simulink model "vd_controller_E9"  (R2017b)
settings: configuration reference "E9_ECU_Configuration" (kept outside this file)
undefined symbols (not defined in the file or in its folder): activate_TC_forMinimal_pTC, ConstantSlipPercent_XCP_pTC, DifferentTorqueFrontAxis_tc, disable_9D_front, disable_9D_rear, disable_slipanglesensor, DiscIntNeverNeededParam, Fz0, lambda_mux_switch_over_XCP_pTC, lambda_mux_XCP_pTC, Lyap_kp_switch_over_XCP_pTC, Lyap_kp_XCP_pTC, Lyap_p, Lyap_TCint, LyapDiscFilter, lyapFilterCoeff_switch_over_XCP_pTC, lyapFilterCoeff_XCP_pTC, mask_SelectInput_pGL, p_Dx1, p_Dx2, Slip_switch_over_XCP_pTC, Sq_PosBadGradient, Sq_PosIsFrozen, Sq_PosOutOfBounds, tire_r_dyn, velLimitInput_switch_over_XCP_pTC, velLimitInput_XCP_pTC, WheelInertia
libraries: SignalProcessingLib x37, simulink x30, hdlsllib x3
(part 2 of 2)

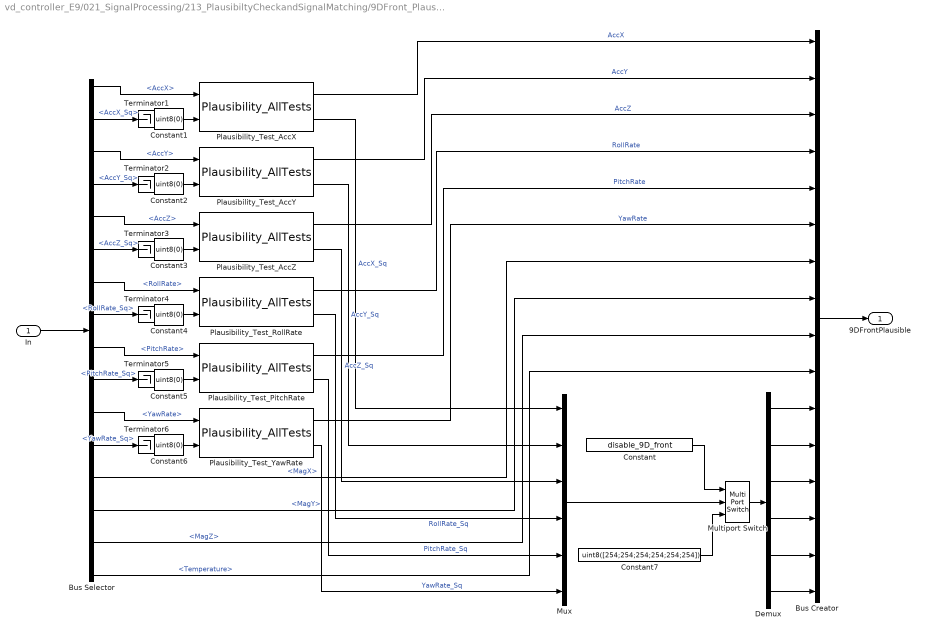
== system vd_controller_E9/021_SignalProcessing/213_PlausibiltyCheckandSignalMatching/9DFront_Plausibility ==
  In : Inport  OutDataTypeStr=Bus: control_9D
  Bus Creator : BusCreator  Inputs=16  OutDataTypeStr=Bus: control_9D
  Bus Selector : BusSelector  OutputSignals=AccX,AccX_Sq,AccY,AccY_Sq,AccZ,AccZ_Sq,RollRate,RollRate_Sq,PitchRate,PitchRate_Sq,YawRate,YawRate_Sq,MagX,MagY,MagZ,Temperature
  Constant : Constant  Value=disable_9D_front
  Constant{1..6} (6 alike) : Constant  Value=uint8(0)
  Constant7 : Constant  Value=uint8([254;254;254;254;254;254])
  Demux : Demux  Outputs=6
  Multiport Switch : MultiPortSwitch  DataPortOrder=Zero-based contiguous  Inputs=2
  Mux : Mux  Inputs=6
  Plausibility_Test_AccX : SignalProcessingLib/Plausibility_AllTests  alpha=0.3  checkGradient=off  deviation=0  threshold=0  alpha2=0  increasingPercentage=0  signalBounds=1e-8  stepDelay=25  upperBound=50  lowerBound=-50  useAlternativeValue=off  useManualAlternativeValue=off  manualAlternativeValue=0
  Plausibility_Test_AccY : SignalProcessingLib/Plausibility_AllTests  alpha=0.3  checkGradient=off  deviation=0  threshold=0  alpha2=0  increasingPercentage=0  signalBounds=1e-8  stepDelay=25  upperBound=50  lowerBound=-50  useAlternativeValue=off  useManualAlternativeValue=off  manualAlternativeValue=0
  Plausibility_Test_AccZ : SignalProcessingLib/Plausibility_AllTests  alpha=0.3  checkGradient=off  deviation=0  threshold=0  alpha2=0  increasingPercentage=0  signalBounds=1e-8  stepDelay=25  upperBound=50  lowerBound=-50  useAlternativeValue=off  useManualAlternativeValue=off  manualAlternativeValue=0
  Plausibility_Test_PitchRate : SignalProcessingLib/Plausibility_AllTests  alpha=0.3  checkGradient=off  deviation=0  threshold=0  alpha2=0  increasingPercentage=0  signalBounds=1e-8  stepDelay=25  upperBound=1.6  lowerBound=-1.6  useAlternativeValue=off  useManualAlternativeValue=off  manualAlternativeValue=0
  Plausibility_Test_RollRate : SignalProcessingLib/Plausibility_AllTests  alpha=0.3  checkGradient=off  deviation=0  threshold=0  alpha2=0  increasingPercentage=0  signalBounds=1e-8  stepDelay=25  upperBound=1.6  lowerBound=-1.6  useAlternativeValue=off  useManualAlternativeValue=off  manualAlternativeValue=0
  Plausibility_Test_YawRate : SignalProcessingLib/Plausibility_AllTests  alpha=0.3  checkGradient=off  deviation=0  threshold=0  alpha2=0  increasingPercentage=0  signalBounds=1e-8  stepDelay=25  upperBound=3  lowerBound=-3  useAlternativeValue=off  useManualAlternativeValue=off  manualAlternativeValue=0
  Terminator{1..6} (6 alike) : Terminator
  9DFrontPlausible : Outport
  wires:
  Plausibility_Test_AccY/1 -> Bus Creator/2  "AccY"
  Bus Selector/3 -> Plausibility_Test_AccY/1  "<AccY>"
  In/1 -> Bus Selector/1
  Plausibility_Test_AccX/1 -> Bus Creator/1  "AccX"
  Bus Selector/1 -> Plausibility_Test_AccX/1  "<AccX>"
  Plausibility_Test_AccZ/1 -> Bus Creator/3  "AccZ"
  Bus Selector/5 -> Plausibility_Test_AccZ/1  "<AccZ>"
  Bus Selector/7 -> Plausibility_Test_RollRate/1  "<RollRate>"
  Plausibility_Test_RollRate/1 -> Bus Creator/4  "RollRate"
  Bus Creator/1 -> 9DFrontPlausible/1
  Plausibility_Test_PitchRate/1 -> Bus Creator/5  "PitchRate"
  Plausibility_Test_YawRate/1 -> Bus Creator/6  "YawRate"
  Bus Selector/9 -> Plausibility_Test_PitchRate/1  "<PitchRate>"
  Bus Selector/11 -> Plausibility_Test_YawRate/1  "<YawRate>"
  Plausibility_Test_YawRate/2 -> Mux/6  "YawRate_Sq"
  Plausibility_Test_PitchRate/2 -> Mux/5  "PitchRate_Sq"
  Plausibility_Test_RollRate/2 -> Mux/4  "RollRate_Sq"
  Plausibility_Test_AccZ/2 -> Mux/3  "AccZ_Sq"
  Bus Selector/13 -> Bus Creator/7  "<MagX>"
  Bus Selector/14 -> Bus Creator/8  "<MagY>"
  Bus Selector/15 -> Bus Creator/9  "<MagZ>"
  Bus Selector/16 -> Bus Creator/10  "<Temperature>"
  Plausibility_Test_AccX/2 -> Mux/1  "AccX_Sq"
  Plausibility_Test_AccY/2 -> Mux/2  "AccY_Sq"
  Constant1/1 -> Plausibility_Test_AccX/2
  Bus Selector/2 -> Terminator1/1  "<AccX_Sq>"
  Constant2/1 -> Plausibility_Test_AccY/2
  Bus Selector/4 -> Terminator2/1  "<AccY_Sq>"
  Constant3/1 -> Plausibility_Test_AccZ/2
  Bus Selector/6 -> Terminator3/1  "<AccZ_Sq>"
  Constant4/1 -> Plausibility_Test_RollRate/2
  Bus Selector/8 -> Terminator4/1  "<RollRate_Sq>"
  Constant5/1 -> Plausibility_Test_PitchRate/2
  Bus Selector/10 -> Terminator5/1  "<PitchRate_Sq>"
  Constant6/1 -> Plausibility_Test_YawRate/2
  Bus Selector/12 -> Terminator6/1  "<YawRate_Sq>"
  Mux/1 -> Multiport Switch/2
  Constant7/1 -> Multiport Switch/3
  Multiport Switch/1 -> Demux/1
  Constant/1 -> Multiport Switch/1
  Demux/1 -> Bus Creator/11
  Demux/2 -> Bus Creator/12
  Demux/3 -> Bus Creator/13
  Demux/4 -> Bus Creator/14
  Demux/5 -> Bus Creator/15
  Demux/6 -> Bus Creator/16

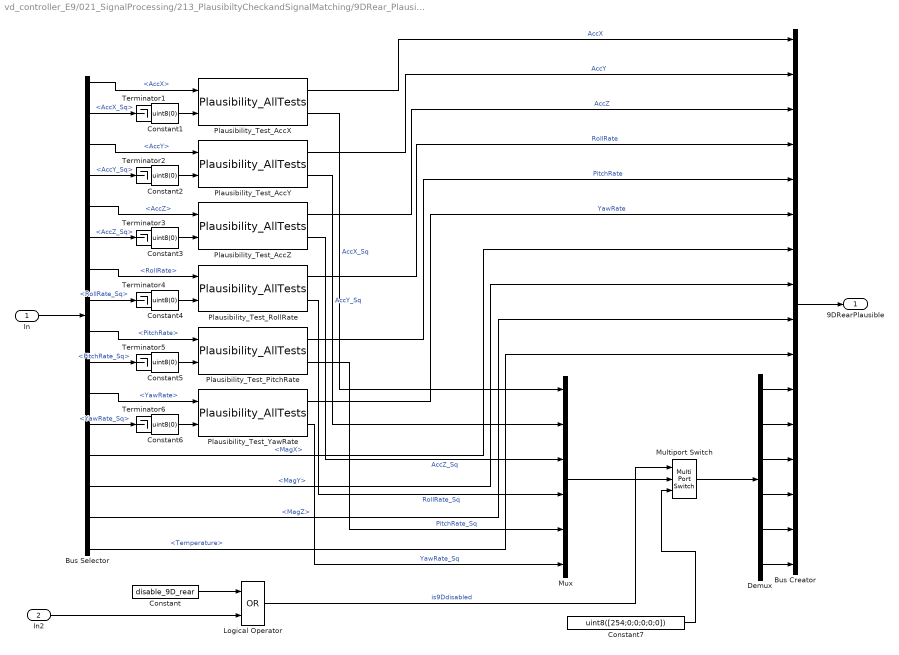
== system vd_controller_E9/021_SignalProcessing/213_PlausibiltyCheckandSignalMatching/9DRear_Plausibility ==
  In : Inport  OutDataTypeStr=Bus: control_9D
  In2 : Inport  Port=2
  Bus Creator : BusCreator  Inputs=16  OutDataTypeStr=Bus: control_9D
  Bus Selector : BusSelector  OutputSignals=AccX,AccX_Sq,AccY,AccY_Sq,AccZ,AccZ_Sq,RollRate,RollRate_Sq,PitchRate,PitchRate_Sq,YawRate,YawRate_Sq,MagX,MagY,MagZ,Temperature
  Constant : Constant  Value=disable_9D_rear
  Constant{1..6} (6 alike) : Constant  Value=uint8(0)
  Constant7 : Constant  Value=uint8([254;0;0;0;0;0])
  Demux : Demux  Outputs=6
  Logical Operator : Logic  Operator=OR  AllPortsSameDT=off  OutDataTypeStr=boolean
  Multiport Switch : MultiPortSwitch  DataPortOrder=Zero-based contiguous  Inputs=2
  Mux : Mux  Inputs=6
  Plausibility_Test_AccX : SignalProcessingLib/Plausibility_AllTests  alpha=0.3  checkGradient=off  deviation=0  threshold=0  alpha2=0  increasingPercentage=0  signalBounds=1e-8  stepDelay=25  upperBound=50  lowerBound=-50  useAlternativeValue=off  useManualAlternativeValue=off  manualAlternativeValue=0
  Plausibility_Test_AccY : SignalProcessingLib/Plausibility_AllTests  alpha=0.3  checkGradient=off  deviation=0  threshold=0  alpha2=0  increasingPercentage=0  signalBounds=1e-8  stepDelay=25  upperBound=50  lowerBound=-50  useAlternativeValue=off  useManualAlternativeValue=off  manualAlternativeValue=0
  Plausibility_Test_AccZ : SignalProcessingLib/Plausibility_AllTests  alpha=0.3  checkGradient=off  deviation=0  threshold=0  alpha2=0  increasingPercentage=0  signalBounds=1e-8  stepDelay=25  upperBound=50  lowerBound=-50  useAlternativeValue=off  useManualAlternativeValue=off  manualAlternativeValue=0
  Plausibility_Test_PitchRate : SignalProcessingLib/Plausibility_AllTests  alpha=0.3  checkGradient=off  deviation=0  threshold=0  alpha2=0  increasingPercentage=0  signalBounds=1e-8  stepDelay=25  upperBound=1.6  lowerBound=-1.6  useAlternativeValue=off  useManualAlternativeValue=off  manualAlternativeValue=0
  Plausibility_Test_RollRate : SignalProcessingLib/Plausibility_AllTests  alpha=0.3  checkGradient=off  deviation=0  threshold=0  alpha2=0  increasingPercentage=0  signalBounds=1e-8  stepDelay=25  upperBound=1.6  lowerBound=-1.6  useAlternativeValue=off  useManualAlternativeValue=off  manualAlternativeValue=0
  Plausibility_Test_YawRate : SignalProcessingLib/Plausibility_AllTests  alpha=0.3  checkGradient=off  deviation=0  threshold=0  alpha2=0  increasingPercentage=0  signalBounds=1e-8  stepDelay=25  upperBound=3  lowerBound=-3  useAlternativeValue=off  useManualAlternativeValue=off  manualAlternativeValue=0
  Terminator{1..6} (6 alike) : Terminator
  9DRearPlausible : Outport
  wires:
  Plausibility_Test_AccY/1 -> Bus Creator/2  "AccY"
  Bus Selector/16 -> Bus Creator/10  "<Temperature>"
  Bus Selector/13 -> Bus Creator/7  "<MagX>"
  Plausibility_Test_YawRate/1 -> Bus Creator/6  "YawRate"
  Bus Selector/15 -> Bus Creator/9  "<MagZ>"
  Plausibility_Test_RollRate/1 -> Bus Creator/4  "RollRate"
  Bus Creator/1 -> 9DRearPlausible/1
  Bus Selector/7 -> Plausibility_Test_RollRate/1  "<RollRate>"
  Bus Selector/5 -> Plausibility_Test_AccZ/1  "<AccZ>"
  Bus Selector/11 -> Plausibility_Test_YawRate/1  "<YawRate>"
  In/1 -> Bus Selector/1
  Plausibility_Test_AccZ/1 -> Bus Creator/3  "AccZ"
  Plausibility_Test_PitchRate/1 -> Bus Creator/5  "PitchRate"
  Plausibility_Test_AccX/1 -> Bus Creator/1  "AccX"
  Bus Selector/1 -> Plausibility_Test_AccX/1  "<AccX>"
  Bus Selector/3 -> Plausibility_Test_AccY/1  "<AccY>"
  Bus Selector/2 -> Terminator1/1  "<AccX_Sq>"
  Plausibility_Test_AccZ/2 -> Mux/3  "AccZ_Sq"
  Plausibility_Test_AccY/2 -> Mux/2  "AccY_Sq"
  Plausibility_Test_PitchRate/2 -> Mux/5  "PitchRate_Sq"
  Bus Selector/14 -> Bus Creator/8  "<MagY>"
  Plausibility_Test_AccX/2 -> Mux/1  "AccX_Sq"
  Plausibility_Test_YawRate/2 -> Mux/6  "YawRate_Sq"
  Plausibility_Test_RollRate/2 -> Mux/4  "RollRate_Sq"
  Bus Selector/9 -> Plausibility_Test_PitchRate/1  "<PitchRate>"
  Constant1/1 -> Plausibility_Test_AccX/2
  Constant2/1 -> Plausibility_Test_AccY/2
  Bus Selector/4 -> Terminator2/1  "<AccY_Sq>"
  Constant3/1 -> Plausibility_Test_AccZ/2
  Bus Selector/6 -> Terminator3/1  "<AccZ_Sq>"
  Constant4/1 -> Plausibility_Test_RollRate/2
  Bus Selector/8 -> Terminator4/1  "<RollRate_Sq>"
  Constant5/1 -> Plausibility_Test_PitchRate/2
  Bus Selector/10 -> Terminator5/1  "<PitchRate_Sq>"
  Constant6/1 -> Plausibility_Test_YawRate/2
  Bus Selector/12 -> Terminator6/1  "<YawRate_Sq>"
  Constant7/1 -> Multiport Switch/3
  Constant/1 -> Logical Operator/1
  Mux/1 -> Multiport Switch/2
  Multiport Switch/1 -> Demux/1
  Demux/6 -> Bus Creator/16
  Demux/5 -> Bus Creator/15
  Demux/4 -> Bus Creator/14
  Demux/3 -> Bus Creator/13
  Demux/2 -> Bus Creator/12
  Demux/1 -> Bus Creator/11
  Logical Operator/1 -> Multiport Switch/1  "is9Ddisabled"
  In2/1 -> Logical Operator/2

== system vd_controller_E9/021_SignalProcessing/213_PlausibiltyCheckandSignalMatching/DriverInput ==
  note: Der DrivingMode aus Inport 2 ist der, der beim Start ausgewählr wurde. Dieser wurde beim E9 in dem Block InverterInControl bestimmt und lässt sich während der Fahrt nicht ändern. Früher in die Funktionsstruktur integreireren, da so weniger umständlich.
  DriverInput_in : Inport
  DrivingMode : Inport  Port=2
  Bus Creator : BusCreator  Inputs=9
  Bus Selector : BusSelector  OutputSignals=db_PTM,db_button_low,vd_button_1,vd_button_2,vd_turnbutton_1,vd_turnbutton_2,driver,DriverInput_Sq
  DriverInput : Outport
  wires:
  DriverInput_in/1 -> Bus Selector/1
  Bus Creator/1 -> DriverInput/1  "DriverInput"
  Bus Selector/1 -> Bus Creator/1  "<db_PTM>"
  Bus Selector/2 -> Bus Creator/2  "<db_button_low>"
  Bus Selector/3 -> Bus Creator/3  "<vd_button_1>"
  Bus Selector/4 -> Bus Creator/4  "<vd_button_2>"
  Bus Selector/5 -> Bus Creator/5  "<vd_turnbutton_1>"
  Bus Selector/6 -> Bus Creator/6  "<vd_turnbutton_2>"
  Bus Selector/7 -> Bus Creator/7  "<driver>"
  DrivingMode/1 -> Bus Creator/9
  Bus Selector/8 -> Bus Creator/8  "<DriverInput_Sq>"

== system vd_controller_E9/021_SignalProcessing/213_PlausibiltyCheckandSignalMatching/DriverRequest_Plausibility ==
  In : Inport  OutDataTypeStr=Bus: control_DriverRequest
  Bus Creator : BusCreator  Inputs=11  OutDataTypeStr=Bus: control_DriverRequest
      settings: InheritFromInputs=off
  Bus Selector : BusSelector  OutputSignals=Pedal_BrakeMech_Value,Pedal_BrakeRecu_Value,SteeringwheelAngle,Pedal_Accel_Value,Pedal_TorqueValid_flag,Pedal_BrakeHard_flag,Pedal_BrakeMech_flag,SteeringValid_flag,Pedal_BrakeValid_flag,SteeringwheelAngle_Sq,Pedal_Accel_Value_Sq
  Data Type Conversion{1..3,6} (4 alike) : DataTypeConversion  OutDataTypeStr=uint8
  Data Type Conversion{4..5,7,9} (4 alike) : DataTypeConversion  OutDataTypeStr=single
  Plausibility_Test_AcceleratorPedal : SignalProcessingLib/Plausibility_AllTests  alpha=0.3  checkGradient=off  deviation=0  threshold=0  alpha2=0  increasingPercentage=0  signalBounds=1e-10  stepDelay=40  upperBound=1  lowerBound=0  useAlternativeValue=off  useManualAlternativeValue=off  manualAlternativeValue=0
  Plausibility_Test_SteeringwheelAngle : SignalProcessingLib/Plausibility_AllTests  alpha=0.3  checkGradient=off  deviation=0  threshold=0  alpha2=0  increasingPercentage=0  signalBounds=1e-10  stepDelay=40  upperBound=120  lowerBound=-120  useAlternativeValue=off  useManualAlternativeValue=off  manualAlternativeValue=0
  DriverRequest : Outport
  wires:
  In/1 -> Bus Selector/1
  Bus Creator/1 -> DriverRequest/1
  Bus Selector/1 -> Data Type Conversion7/1  "<Pedal_BrakeMech_Value>"
  Bus Selector/2 -> Data Type Conversion5/1  "<Pedal_BrakeRecu_Value>"
  Bus Selector/3 -> Plausibility_Test_SteeringwheelAngle/1  "<SteeringwheelAngle>"
  Plausibility_Test_SteeringwheelAngle/1 -> Data Type Conversion4/1  "SteeringwheelAngle"
  Bus Selector/4 -> Plausibility_Test_AcceleratorPedal/1  "<Pedal_Accel_Value>"
  Bus Selector/5 -> Bus Creator/5  "<Pedal_TorqueValid_flag>"
  Bus Selector/6 -> Bus Creator/6  "<Pedal_BrakeHard_flag>"
  Bus Selector/7 -> Bus Creator/7  "<Pedal_BrakeMech_flag>"
  Bus Selector/8 -> Bus Creator/8  "<SteeringValid_flag>"
  Bus Selector/9 -> Bus Creator/9  "<Pedal_BrakeValid_flag>"
  Plausibility_Test_SteeringwheelAngle/2 -> Data Type Conversion3/1  "SteeringwheelAngle_Sq"
  Plausibility_Test_AcceleratorPedal/1 -> Data Type Conversion9/1  "Pedal_Accel_Value"
  Bus Selector/10 -> Data Type Conversion6/1  "<SteeringwheelAngle_Sq>"
  Data Type Conversion7/1 -> Bus Creator/1
  Data Type Conversion5/1 -> Bus Creator/2
  Data Type Conversion4/1 -> Bus Creator/3
  Data Type Conversion9/1 -> Bus Creator/4
  Bus Selector/11 -> Data Type Conversion1/1  "<Pedal_Accel_Value_Sq>"
  Plausibility_Test_AcceleratorPedal/2 -> Data Type Conversion2/1  "Pedal_Accel_Value_Sq"
  Data Type Conversion2/1 -> Bus Creator/11
  Data Type Conversion6/1 -> Plausibility_Test_SteeringwheelAngle/2
  Data Type Conversion1/1 -> Plausibility_Test_AcceleratorPedal/2
  Data Type Conversion3/1 -> Bus Creator/10

== system vd_controller_E9/021_SignalProcessing/213_PlausibiltyCheckandSignalMatching/Electric_Plausibility ==
  In : Inport  OutDataTypeStr=Bus: control_Electric
  Bus Creator : BusCreator  Inputs=12  OutDataTypeStr=Bus: control_Electric
  Bus Selector : BusSelector  OutputSignals=BatSOC,BatVoltage,BatPower,BatCurrent,AvgCellVoltage,MaxCellVoltage,MinCellVoltage,IVTEnergy,MinCellTemp,IVT_VoltageCurrent_Sq,IVT_Energy_Sq,HVM_BMS_Sq
  Data Type Conversion22 : DataTypeConversion  OutDataTypeStr=single
  Plausibility_Test_IVTEnergy : SignalProcessingLib/Plausibility_AllTests  alpha=0.5  checkGradient=off  deviation=0  threshold=0  alpha2=0  increasingPercentage=0  signalBounds=1e-10  stepDelay=40  upperBound=120000  lowerBound=-120000  useAlternativeValue=off  useManualAlternativeValue=off  manualAlternativeValue=0
  ElectricPlausible : Outport
  wires:
  Bus Selector/8 -> Plausibility_Test_IVTEnergy/1  "<IVTEnergy>"
  Bus Selector/7 -> Bus Creator/7  "<MinCellVoltage>"
  In/1 -> Bus Selector/1
  Bus Creator/1 -> ElectricPlausible/1  "Electric"
  Bus Selector/1 -> Bus Creator/1  "<BatSOC>"
  Bus Selector/2 -> Bus Creator/2  "<BatVoltage>"
  Bus Selector/3 -> Bus Creator/3  "<BatPower>"
  Bus Selector/4 -> Bus Creator/4  "<BatCurrent>"
  Bus Selector/5 -> Bus Creator/5  "<AvgCellVoltage>"
  Bus Selector/6 -> Bus Creator/6  "<MaxCellVoltage>"
  Bus Selector/9 -> Bus Creator/9  "<MinCellTemp>"
  Bus Selector/10 -> Bus Creator/10  "<IVT_VoltageCurrent_Sq>"
  Bus Selector/11 -> Plausibility_Test_IVTEnergy/2  "<IVT_Energy_Sq>"
  Bus Selector/12 -> Bus Creator/12  "<HVM_BMS_Sq>"
  Plausibility_Test_IVTEnergy/2 -> Bus Creator/11  "IVTEnergy_Sq"
  Plausibility_Test_IVTEnergy/1 -> Data Type Conversion22/1  "IVTEnergy"
  Data Type Conversion22/1 -> Bus Creator/8

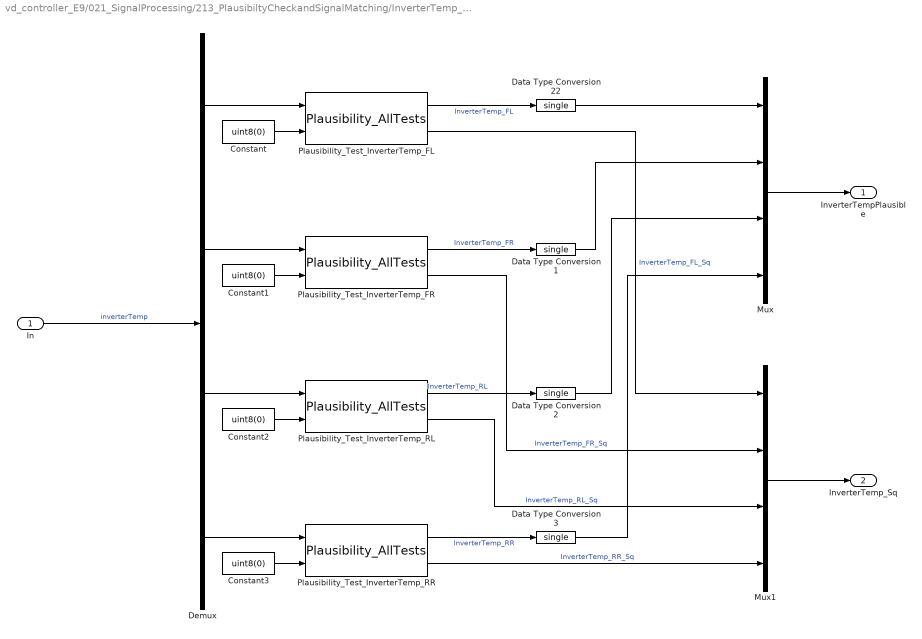
== system vd_controller_E9/021_SignalProcessing/213_PlausibiltyCheckandSignalMatching/InverterTemp_Plausibility ==
  In : Inport  OutDataTypeStr=single  PortDimensions=4
  Constant{,1..3} (4 alike) : Constant  Value=uint8(0)
  Data Type Conversion{1..3,22} (4 alike) : DataTypeConversion  OutDataTypeStr=single
  Demux : Demux
  Mux : Mux
  Mux1 : Mux
  Plausibility_Test_InverterTemp_FL : SignalProcessingLib/Plausibility_AllTests  alpha=0  checkGradient=off  deviation=0  threshold=0  alpha2=0  increasingPercentage=0  signalBounds=1e-12  stepDelay=40  upperBound=75  lowerBound=-10  useAlternativeValue=off  useManualAlternativeValue=off  manualAlternativeValue=0
  Plausibility_Test_InverterTemp_FR : SignalProcessingLib/Plausibility_AllTests  alpha=0.5  checkGradient=off  deviation=0  threshold=0  alpha2=0  increasingPercentage=0  signalBounds=1e-12  stepDelay=40  upperBound=75  lowerBound=-10  useAlternativeValue=off  useManualAlternativeValue=off  manualAlternativeValue=0
  Plausibility_Test_InverterTemp_RL : SignalProcessingLib/Plausibility_AllTests  alpha=0.5  checkGradient=off  deviation=0  threshold=0  alpha2=0  increasingPercentage=0  signalBounds=1e-12  stepDelay=40  upperBound=75  lowerBound=-10  useAlternativeValue=off  useManualAlternativeValue=off  manualAlternativeValue=0
  Plausibility_Test_InverterTemp_RR : SignalProcessingLib/Plausibility_AllTests  alpha=0.5  checkGradient=off  deviation=0  threshold=0  alpha2=0  increasingPercentage=0  signalBounds=1e-12  stepDelay=40  upperBound=75  lowerBound=-10  useAlternativeValue=off  useManualAlternativeValue=off  manualAlternativeValue=0
  InverterTempPlausible : Outport
  InverterTemp_Sq : Outport  Port=2
  wires:
  Plausibility_Test_InverterTemp_FR/1 -> Data Type Conversion1/1  "InverterTemp_FR"
  In/1 -> Demux/1  "inverterTemp"
  Plausibility_Test_InverterTemp_FL/1 -> Data Type Conversion22/1  "InverterTemp_FL"
  Plausibility_Test_InverterTemp_RL/1 -> Data Type Conversion2/1  "InverterTemp_RL"
  Demux/1 -> Plausibility_Test_InverterTemp_FL/1
  Demux/2 -> Plausibility_Test_InverterTemp_FR/1
  Demux/3 -> Plausibility_Test_InverterTemp_RL/1
  Plausibility_Test_InverterTemp_RL/2 -> Mux1/3  "InverterTemp_RL_Sq"
  Plausibility_Test_InverterTemp_FR/2 -> Mux1/2  "InverterTemp_FR_Sq"
  Demux/4 -> Plausibility_Test_InverterTemp_RR/1
  Constant/1 -> Plausibility_Test_InverterTemp_FL/2
  Constant1/1 -> Plausibility_Test_InverterTemp_FR/2
  Constant2/1 -> Plausibility_Test_InverterTemp_RL/2
  Constant3/1 -> Plausibility_Test_InverterTemp_RR/2
  Plausibility_Test_InverterTemp_RR/1 -> Data Type Conversion3/1  "InverterTemp_RR"
  Mux/1 -> InverterTempPlausible/1
  Mux1/1 -> InverterTemp_Sq/1
  Plausibility_Test_InverterTemp_RR/2 -> Mux1/4  "InverterTemp_RR_Sq"
  Plausibility_Test_InverterTemp_FL/2 -> Mux1/1  "InverterTemp_FL_Sq"
  Data Type Conversion22/1 -> Mux/1
  Data Type Conversion1/1 -> Mux/2
  Data Type Conversion2/1 -> Mux/3
  Data Type Conversion3/1 -> Mux/4

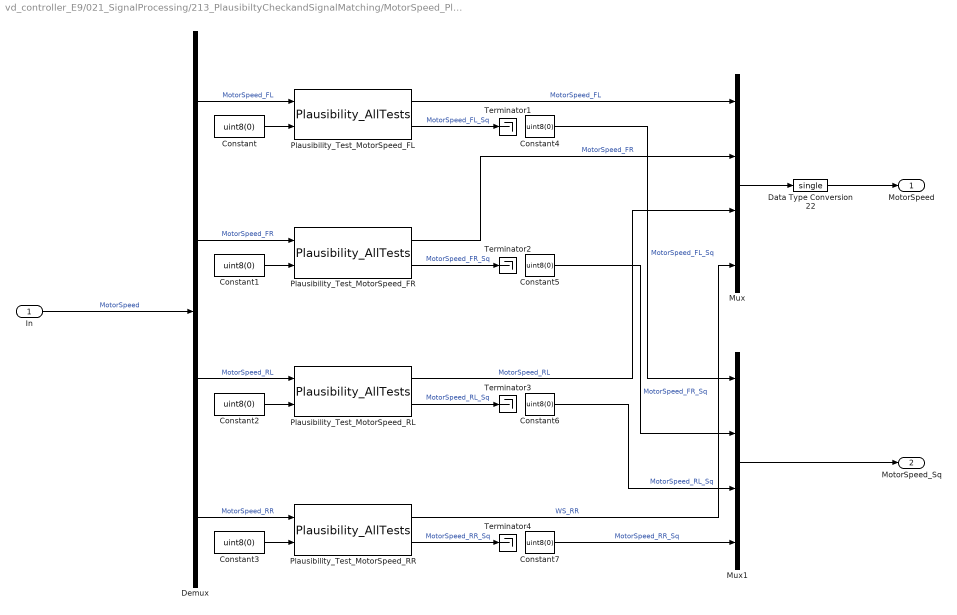
== system vd_controller_E9/021_SignalProcessing/213_PlausibiltyCheckandSignalMatching/MotorSpeed_Plausibility ==
  In : Inport
  Constant{,1..7} (8 alike) : Constant  Value=uint8(0)
  Data Type Conversion22 : DataTypeConversion  OutDataTypeStr=single
  Demux : Demux
  Mux : Mux
  Mux1 : Mux
  Plausibility_Test_MotorSpeed_FL : SignalProcessingLib/Plausibility_AllTests  alpha=0.4  checkGradient=off  deviation=0  threshold=0  alpha2=0  increasingPercentage=0  signalBounds=1e-10  stepDelay=40  upperBound=20000  lowerBound=-10000  useAlternativeValue=off  useManualAlternativeValue=off  manualAlternativeValue=0
  Plausibility_Test_MotorSpeed_FR : SignalProcessingLib/Plausibility_AllTests  alpha=0.4  checkGradient=off  deviation=0  threshold=0  alpha2=0  increasingPercentage=0  signalBounds=1e-10  stepDelay=40  upperBound=20000  lowerBound=-10000  useAlternativeValue=off  useManualAlternativeValue=off  manualAlternativeValue=0
  Plausibility_Test_MotorSpeed_RL : SignalProcessingLib/Plausibility_AllTests  alpha=0.4  checkGradient=off  deviation=0  threshold=0  alpha2=0  increasingPercentage=0  signalBounds=1e-10  stepDelay=40  upperBound=20000  lowerBound=-10000  useAlternativeValue=off  useManualAlternativeValue=off  manualAlternativeValue=0
  Plausibility_Test_MotorSpeed_RR : SignalProcessingLib/Plausibility_AllTests  alpha=0.4  checkGradient=off  deviation=0  threshold=0  alpha2=0  increasingPercentage=0  signalBounds=1e-10  stepDelay=40  upperBound=20000  lowerBound=-10000  useAlternativeValue=off  useManualAlternativeValue=off  manualAlternativeValue=0
  Terminator{1..4} (4 alike) : Terminator
  MotorSpeed : Outport
  MotorSpeed_Sq : Outport  Port=2
  wires:
  Constant4/1 -> Mux1/1  "MotorSpeed_FL_Sq"
  Constant7/1 -> Mux1/4  "MotorSpeed_RR_Sq"
  Mux1/1 -> MotorSpeed_Sq/1
  Mux/1 -> Data Type Conversion22/1
  Plausibility_Test_MotorSpeed_RR/1 -> Mux/4  "WS_RR"
  Constant3/1 -> Plausibility_Test_MotorSpeed_RR/2
  Constant2/1 -> Plausibility_Test_MotorSpeed_RL/2
  Constant1/1 -> Plausibility_Test_MotorSpeed_FR/2
  Constant/1 -> Plausibility_Test_MotorSpeed_FL/2
  Demux/4 -> Plausibility_Test_MotorSpeed_RR/1  "MotorSpeed_RR"
  Constant5/1 -> Mux1/2  "MotorSpeed_FR_Sq"
  Constant6/1 -> Mux1/3  "MotorSpeed_RL_Sq"
  Demux/3 -> Plausibility_Test_MotorSpeed_RL/1  "MotorSpeed_RL"
  Demux/2 -> Plausibility_Test_MotorSpeed_FR/1  "MotorSpeed_FR"
  Demux/1 -> Plausibility_Test_MotorSpeed_FL/1  "MotorSpeed_FL"
  Plausibility_Test_MotorSpeed_RL/1 -> Mux/3  "MotorSpeed_RL"
  Plausibility_Test_MotorSpeed_FL/1 -> Mux/1  "MotorSpeed_FL"
  In/1 -> Demux/1  "MotorSpeed"
  Plausibility_Test_MotorSpeed_FR/1 -> Mux/2  "MotorSpeed_FR"
  Data Type Conversion22/1 -> MotorSpeed/1
  Plausibility_Test_MotorSpeed_FL/2 -> Terminator1/1  "MotorSpeed_FL_Sq"
  Plausibility_Test_MotorSpeed_FR/2 -> Terminator2/1  "MotorSpeed_FR_Sq"
  Plausibility_Test_MotorSpeed_RL/2 -> Terminator3/1  "MotorSpeed_RL_Sq"
  Plausibility_Test_MotorSpeed_RR/2 -> Terminator4/1  "MotorSpeed_RR_Sq"

== system vd_controller_E9/021_SignalProcessing/213_PlausibiltyCheckandSignalMatching/MotorTemp_Plausibility ==
  In : Inport
  Constant{,1..3} (4 alike) : Constant  Value=uint8(0)
  Data Type Conversion{1..3,22} (4 alike) : DataTypeConversion  OutDataTypeStr=single
  Demux : Demux
  Mux : Mux
  Mux1 : Mux
  Plausibility_Test_MotorTemp_FL : SignalProcessingLib/Plausibility_AllTests  alpha=0.5  checkGradient=off  deviation=0  threshold=0  alpha2=0  increasingPercentage=0  signalBounds=1e-12  stepDelay=40  upperBound=1300  lowerBound=-10  useAlternativeValue=off  useManualAlternativeValue=off  manualAlternativeValue=0
  Plausibility_Test_MotorTemp_FR : SignalProcessingLib/Plausibility_AllTests  alpha=0.5  checkGradient=off  deviation=0  threshold=0  alpha2=0  increasingPercentage=0  signalBounds=1e-12  stepDelay=40  upperBound=130  lowerBound=-10  useAlternativeValue=off  useManualAlternativeValue=off  manualAlternativeValue=0
  Plausibility_Test_MotorTemp_RL : SignalProcessingLib/Plausibility_AllTests  alpha=0.5  checkGradient=off  deviation=0  threshold=0  alpha2=0  increasingPercentage=0  signalBounds=1e-12  stepDelay=40  upperBound=130  lowerBound=-10  useAlternativeValue=off  useManualAlternativeValue=off  manualAlternativeValue=0
  Plausibility_Test_MotorTemp_RR : SignalProcessingLib/Plausibility_AllTests  alpha=0.5  checkGradient=off  deviation=0  threshold=0  alpha2=0  increasingPercentage=0  signalBounds=1e-12  stepDelay=40  upperBound=130  lowerBound=-10  useAlternativeValue=off  useManualAlternativeValue=off  manualAlternativeValue=0
  MotorTempPlausible : Outport
  MotorTemp_Sq : Outport  Port=2
  wires:
  Plausibility_Test_MotorTemp_FR/1 -> Data Type Conversion1/1  "MotorTemp_FR"
  In/1 -> Demux/1  "motorTemp"
  Plausibility_Test_MotorTemp_FL/1 -> Data Type Conversion22/1  "MotorTemp_FL"
  Plausibility_Test_MotorTemp_RL/1 -> Data Type Conversion2/1  "MotorTemp_RL"
  Demux/1 -> Plausibility_Test_MotorTemp_FL/1
  Demux/2 -> Plausibility_Test_MotorTemp_FR/1
  Demux/3 -> Plausibility_Test_MotorTemp_RL/1
  Plausibility_Test_MotorTemp_RL/2 -> Mux1/3  "MotorTemp_RL_Sq"
  Plausibility_Test_MotorTemp_FR/2 -> Mux1/2  "MotorTemp_FR_Sq"
  Demux/4 -> Plausibility_Test_MotorTemp_RR/1
  Constant/1 -> Plausibility_Test_MotorTemp_FL/2
  Constant1/1 -> Plausibility_Test_MotorTemp_FR/2
  Constant2/1 -> Plausibility_Test_MotorTemp_RL/2
  Constant3/1 -> Plausibility_Test_MotorTemp_RR/2
  Plausibility_Test_MotorTemp_RR/1 -> Data Type Conversion3/1  "MotorTemp_RR"
  Mux/1 -> MotorTempPlausible/1
  Mux1/1 -> MotorTemp_Sq/1
  Plausibility_Test_MotorTemp_RR/2 -> Mux1/4  "MotorTemp_RR_Sq"
  Plausibility_Test_MotorTemp_FL/2 -> Mux1/1  "MotorTemp_Sq"
  Data Type Conversion22/1 -> Mux/1
  Data Type Conversion1/1 -> Mux/2
  Data Type Conversion2/1 -> Mux/3
  Data Type Conversion3/1 -> Mux/4

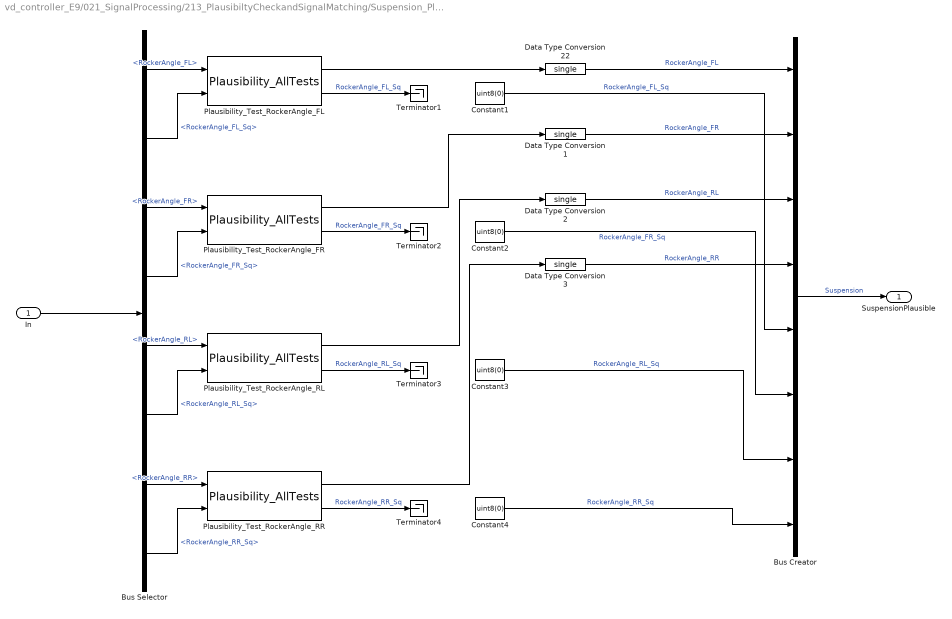
== system vd_controller_E9/021_SignalProcessing/213_PlausibiltyCheckandSignalMatching/Suspension_Plausibility ==
  In : Inport  OutDataTypeStr=Bus: control_Suspension
  Bus Creator : BusCreator  Inputs=8  OutDataTypeStr=Bus: control_Suspension
  Bus Selector : BusSelector  OutputSignals=RockerAngle_FL,RockerAngle_FL_Sq,RockerAngle_FR,RockerAngle_FR_Sq,RockerAngle_RL,RockerAngle_RL_Sq,RockerAngle_RR,RockerAngle_RR_Sq
  Constant{1..4} (4 alike) : Constant  Value=uint8(0)
  Data Type Conversion{1..3,22} (4 alike) : DataTypeConversion  OutDataTypeStr=single
  Plausibility_Test_RockerAngle_FL : SignalProcessingLib/Plausibility_AllTests  alpha=0.5  checkGradient=off  deviation=0  threshold=0  alpha2=0  increasingPercentage=0  signalBounds=1e-10  stepDelay=38  upperBound=30  lowerBound=-30  useAlternativeValue=off  useManualAlternativeValue=off  manualAlternativeValue=0
  Plausibility_Test_RockerAngle_FR : SignalProcessingLib/Plausibility_AllTests  alpha=0.5  checkGradient=off  deviation=0  threshold=0  alpha2=0  increasingPercentage=0  signalBounds=1e-10  stepDelay=38  upperBound=30  lowerBound=-30  useAlternativeValue=off  useManualAlternativeValue=off  manualAlternativeValue=0
  Plausibility_Test_RockerAngle_RL : SignalProcessingLib/Plausibility_AllTests  alpha=0.5  checkGradient=off  deviation=0  threshold=0  alpha2=0  increasingPercentage=0  signalBounds=1e-10  stepDelay=38  upperBound=30  lowerBound=-30  useAlternativeValue=off  useManualAlternativeValue=off  manualAlternativeValue=0
  Plausibility_Test_RockerAngle_RR : SignalProcessingLib/Plausibility_AllTests  alpha=0.5  checkGradient=off  deviation=0  threshold=0  alpha2=0  increasingPercentage=0  signalBounds=1e-10  stepDelay=38  upperBound=30  lowerBound=-30  useAlternativeValue=off  useManualAlternativeValue=off  manualAlternativeValue=0
  Terminator{1..4} (4 alike) : Terminator
  SuspensionPlausible : Outport
  wires:
  Constant1/1 -> Bus Creator/5  "RockerAngle_FL_Sq"
  Constant2/1 -> Bus Creator/6  "RockerAngle_FR_Sq"
  Constant3/1 -> Bus Creator/7  "RockerAngle_RL_Sq"
  Bus Selector/6 -> Plausibility_Test_RockerAngle_RL/2  "<RockerAngle_RL_Sq>"
  Bus Selector/5 -> Plausibility_Test_RockerAngle_RL/1  "<RockerAngle_RL>"
  Bus Selector/4 -> Plausibility_Test_RockerAngle_FR/2  "<RockerAngle_FR_Sq>"
  Bus Selector/3 -> Plausibility_Test_RockerAngle_FR/1  "<RockerAngle_FR>"
  Bus Selector/2 -> Plausibility_Test_RockerAngle_FL/2  "<RockerAngle_FL_Sq>"
  Bus Selector/1 -> Plausibility_Test_RockerAngle_FL/1  "<RockerAngle_FL>"
  Bus Creator/1 -> SuspensionPlausible/1  "Suspension"
  Plausibility_Test_RockerAngle_RL/1 -> Data Type Conversion2/1
  Plausibility_Test_RockerAngle_FL/1 -> Data Type Conversion22/1
  In/1 -> Bus Selector/1
  Plausibility_Test_RockerAngle_FR/1 -> Data Type Conversion1/1
  Bus Selector/7 -> Plausibility_Test_RockerAngle_RR/1  "<RockerAngle_RR>"
  Constant4/1 -> Bus Creator/8  "RockerAngle_RR_Sq"
  Plausibility_Test_RockerAngle_RR/1 -> Data Type Conversion3/1
  Bus Selector/8 -> Plausibility_Test_RockerAngle_RR/2  "<RockerAngle_RR_Sq>"
  Data Type Conversion22/1 -> Bus Creator/1  "RockerAngle_FL"
  Data Type Conversion1/1 -> Bus Creator/2  "RockerAngle_FR"
  Data Type Conversion2/1 -> Bus Creator/3  "RockerAngle_RL"
  Data Type Conversion3/1 -> Bus Creator/4  "RockerAngle_RR"
  Plausibility_Test_RockerAngle_FL/2 -> Terminator1/1  "RockerAngle_FL_Sq"
  Plausibility_Test_RockerAngle_FR/2 -> Terminator2/1  "RockerAngle_FR_Sq"
  Plausibility_Test_RockerAngle_RL/2 -> Terminator3/1  "RockerAngle_RL_Sq"
  Plausibility_Test_RockerAngle_RR/2 -> Terminator4/1  "RockerAngle_RR_Sq"

== system vd_controller_E9/021_SignalProcessing/213_PlausibiltyCheckandSignalMatching/WheelSpeed_Plausibility ==
  note: Dieser Block ist eigentlich überflüssig. Der Zusammenhang von MotorSpeed und WheelSpeed ist sehr simpel (selbe Messgröße).
      | Es reicht aus, nur diePlausibilität von MotorSpeed zu prüfen und daraufhin MotorSpeed und WheelSpeed gleichzeitig zu bewerten.
  In : Inport
  Constant{,1..3} (4 alike) : Constant  Value=uint8(0)
  Data Type Conversion{1..3,22} (4 alike) : DataTypeConversion  OutDataTypeStr=single
  Demux : Demux
  Mux : Mux
  Mux1 : Mux
  Plausibility_Test_WheelSpeed_FL : SignalProcessingLib/Plausibility_AllTests  alpha=0.3  checkGradient=off  deviation=0  threshold=0  alpha2=0  increasingPercentage=0  signalBounds=1e-12  stepDelay=40  upperBound=100  lowerBound=-10  useAlternativeValue=off  useManualAlternativeValue=off  manualAlternativeValue=0
  Plausibility_Test_WheelSpeed_FR : SignalProcessingLib/Plausibility_AllTests  alpha=0.3  checkGradient=off  deviation=0  threshold=0  alpha2=0  increasingPercentage=0  signalBounds=1e-12  stepDelay=40  upperBound=100  lowerBound=-10  useAlternativeValue=off  useManualAlternativeValue=off  manualAlternativeValue=0
  Plausibility_Test_WheelSpeed_RL : SignalProcessingLib/Plausibility_AllTests  alpha=0.3  checkGradient=off  deviation=0  threshold=0  alpha2=0  increasingPercentage=0  signalBounds=1e-12  stepDelay=40  upperBound=100  lowerBound=-10  useAlternativeValue=off  useManualAlternativeValue=off  manualAlternativeValue=0
  Plausibility_Test_WheelSpeed_RR : SignalProcessingLib/Plausibility_AllTests  alpha=0.3  checkGradient=off  deviation=0  threshold=0  alpha2=0  increasingPercentage=0  signalBounds=1e-12  stepDelay=40  upperBound=100  lowerBound=-10  useAlternativeValue=off  useManualAlternativeValue=off  manualAlternativeValue=0
  WheelSpeedPlausible : Outport
  WheelSpeed_Sq : Outport  Port=2
  wires:
  Plausibility_Test_WheelSpeed_FR/1 -> Data Type Conversion1/1  "WheelSpeed_FR"
  In/1 -> Demux/1  "wheelSpeed"
  Plausibility_Test_WheelSpeed_FL/1 -> Data Type Conversion22/1  "WheelSpeed_FL"
  Plausibility_Test_WheelSpeed_RL/1 -> Data Type Conversion2/1  "WheelSpeed_RL"
  Demux/1 -> Plausibility_Test_WheelSpeed_FL/1  "WheelSpeed_FL"
  Demux/2 -> Plausibility_Test_WheelSpeed_FR/1  "WheelSpeed_FR"
  Demux/3 -> Plausibility_Test_WheelSpeed_RL/1  "WheelSpeed_RL"
  Plausibility_Test_WheelSpeed_RL/2 -> Mux1/3  "WheelSpeed_RL_Sq"
  Plausibility_Test_WheelSpeed_FR/2 -> Mux1/2  "WheelSpeed_FR_Sq"
  Demux/4 -> Plausibility_Test_WheelSpeed_RR/1  "WheelSpeed_RR"
  Constant/1 -> Plausibility_Test_WheelSpeed_FL/2
  Constant1/1 -> Plausibility_Test_WheelSpeed_FR/2
  Constant2/1 -> Plausibility_Test_WheelSpeed_RL/2
  Constant3/1 -> Plausibility_Test_WheelSpeed_RR/2
  Plausibility_Test_WheelSpeed_RR/1 -> Data Type Conversion3/1  "WheelSpeed_RR"
  Mux/1 -> WheelSpeedPlausible/1
  Mux1/1 -> WheelSpeed_Sq/1
  Plausibility_Test_WheelSpeed_RR/2 -> Mux1/4  "WheelSpeed_RR_Sq"
  Plausibility_Test_WheelSpeed_FL/2 -> Mux1/1  "WheelSpeed_FL_Sq"
  Data Type Conversion22/1 -> Mux/1
  Data Type Conversion1/1 -> Mux/2
  Data Type Conversion2/1 -> Mux/3
  Data Type Conversion3/1 -> Mux/4

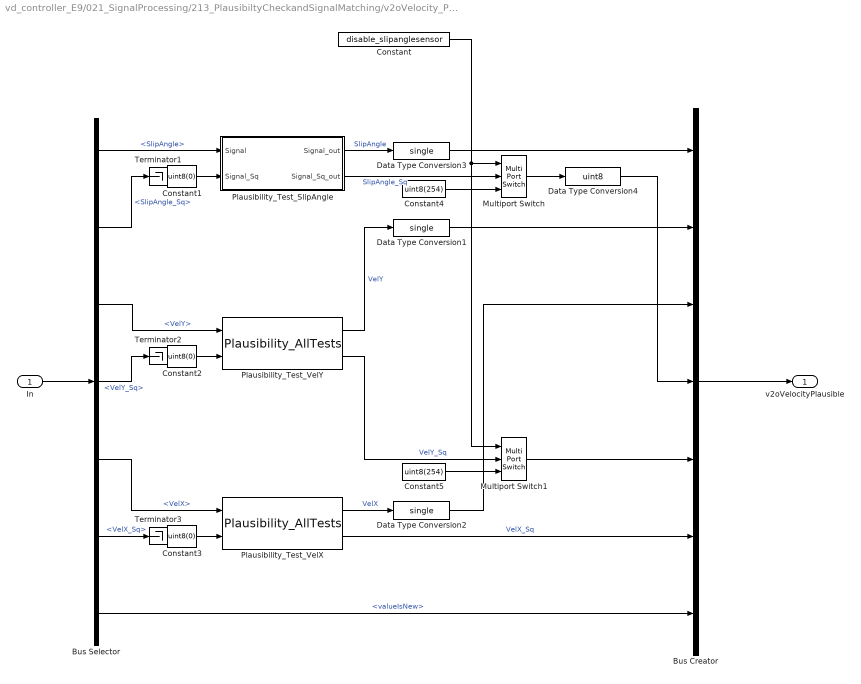
== system vd_controller_E9/021_SignalProcessing/213_PlausibiltyCheckandSignalMatching/v2oVelocity_Plausibility ==
  In : Inport  OutDataTypeStr=Bus: control_Velocity
  Bus Creator : BusCreator  Inputs=7  OutDataTypeStr=Bus: control_Velocity
  Bus Selector : BusSelector  OutputSignals=SlipAngle,SlipAngle_Sq,VelY,VelY_Sq,VelX,VelX_Sq,valueIsNew
  Constant : Constant  Value=disable_slipanglesensor
  Constant1 : Constant  Value=uint8(0)
  Constant2 : Constant  Value=uint8(0)
  Constant3 : Constant  Value=uint8(0)
  Constant4 : Constant  Value=uint8(254)
  Constant5 : Constant  Value=uint8(254)
  Data Type Conversion1 : DataTypeConversion  OutDataTypeStr=single
  Data Type Conversion2 : DataTypeConversion  OutDataTypeStr=single
  Data Type Conversion3 : DataTypeConversion  OutDataTypeStr=single
  Data Type Conversion4 : DataTypeConversion  OutDataTypeStr=uint8
  Multiport Switch : MultiPortSwitch  DataPortOrder=Zero-based contiguous  Inputs=2
  Multiport Switch1 : MultiPortSwitch  DataPortOrder=Zero-based contiguous  Inputs=2
  Plausibility_Test_SlipAngle : Subsystem  AncestorBlock=SignalProcessingLib/Plausibility_AllTests  mask{alpha=0.3, checkGradient=off, deviation=0, threshold=0, alpha2=0, increasingPercentage=0, signalBounds=1e-8, stepDelay=35, upperBound=90, lowerBound=-90, useAlternativeValue=off, useManualAlternativeValue=off, manualAlternativeValue=0}
      mask prompts: alpha "alpha-value"; checkGradient "Shall the gradient be controlled?"; deviation "gain for accepted deviation"; threshold "Maximal Change per Second"; alpha2 "Inertia of mean (0-1)"; increasingPercentage "percent of the max. changerate add to the allowed deviation [%]"; signalBounds "Signal Bounds"; stepDelay "Step Delay"; upperBound "upper bound"; lowerBound "lower bound"; useAlternativeValue "Shall a alternative value be used if signal is not plausible?"; useManualAlternativeValue "Shall a manually given Value be used? Otherwise signal is held."; manualAlternativeValue "manually given Value"
      mask DialogControl LowPassSettings Prompt: lowpass
      mask DialogControl BadGradientSettings Prompt: bad gradient
      mask DialogControl increasingPercentage Tooltip: How many percent of the max. Change per Second the allowed deviation rises
      mask DialogControl Container8 Prompt: frozen value
      mask DialogControl signalBounds Tooltip: (in which bounds consecutive singals can differ to be detected as frozen )
      mask DialogControl stepDelay Tooltip: how many steps the singal must be within the bounds, so that the signal is detected as frozen
      mask DialogControl Bounds Prompt: bounds
      mask DialogControl AlternativeValue Prompt: alternative Value
      mask DialogControl Container12 Prompt: Use manually given Value
  Plausibility_Test_VelX : SignalProcessingLib/Plausibility_AllTests  alpha=0.5  checkGradient=off  deviation=0  threshold=0  alpha2=0  increasingPercentage=0  signalBounds=1e-8  stepDelay=35  upperBound=35  lowerBound=-3  useAlternativeValue=off  useManualAlternativeValue=off  manualAlternativeValue=0
  Plausibility_Test_VelY : SignalProcessingLib/Plausibility_AllTests  alpha=0.5  checkGradient=off  deviation=0  threshold=0  alpha2=0  increasingPercentage=0  signalBounds=1e-8  stepDelay=35  upperBound=50  lowerBound=-50  useAlternativeValue=off  useManualAlternativeValue=off  manualAlternativeValue=0
  Terminator1 : Terminator
  Terminator2 : Terminator
  Terminator3 : Terminator
  v2oVelocityPlausible : Outport
  wires:
  Plausibility_Test_VelY/1 -> Data Type Conversion1/1  "VelY"
  In/1 -> Bus Selector/1
  Plausibility_Test_SlipAngle/1(Signal_out) -> Data Type Conversion3/1  "SlipAngle"
  Plausibility_Test_VelX/1 -> Data Type Conversion2/1  "VelX"
  Bus Creator/1 -> v2oVelocityPlausible/1
  Bus Selector/1 -> Plausibility_Test_SlipAngle/1(Signal)  "<SlipAngle>"
  Bus Selector/2 -> Terminator1/1  "<SlipAngle_Sq>"
  Bus Selector/3 -> Plausibility_Test_VelY/1  "<VelY>"
  Bus Selector/4 -> Terminator2/1  "<VelY_Sq>"
  Bus Selector/5 -> Plausibility_Test_VelX/1  "<VelX>"
  Bus Selector/6 -> Terminator3/1  "<VelX_Sq>"
  Bus Selector/7 -> Bus Creator/7  "<valueIsNew>"
  Data Type Conversion1/1 -> Bus Creator/2
  Data Type Conversion3/1 -> Bus Creator/1
  Data Type Conversion2/1 -> Bus Creator/3
  Plausibility_Test_SlipAngle/2(Signal_Sq_out) -> Multiport Switch/2  "SlipAngle_Sq"
  Plausibility_Test_VelY/2 -> Multiport Switch1/2  "VelY_Sq"
  Plausibility_Test_VelX/2 -> Bus Creator/6  "VelX_Sq"
  Constant1/1 -> Plausibility_Test_SlipAngle/2(Signal_Sq)
  Constant2/1 -> Plausibility_Test_VelY/2
  Constant3/1 -> Plausibility_Test_VelX/2
  Constant/1 -> Multiport Switch1/1, Multiport Switch/1
  Multiport Switch/1 -> Data Type Conversion4/1
  Constant4/1 -> Multiport Switch/3
  Multiport Switch1/1 -> Bus Creator/5
  Constant5/1 -> Multiport Switch1/3
  Data Type Conversion4/1 -> Bus Creator/4

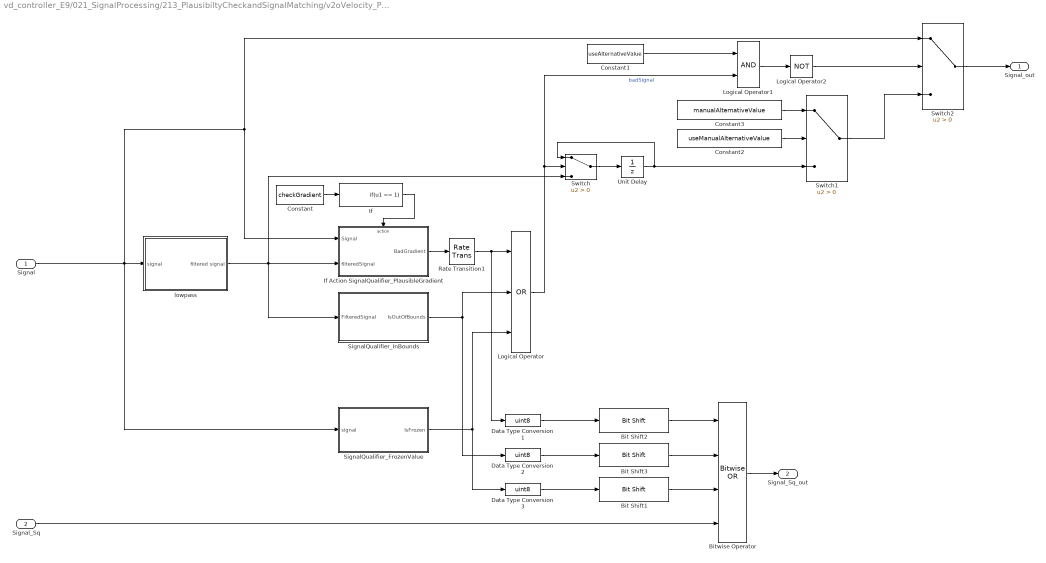
== system vd_controller_E9/021_SignalProcessing/213_PlausibiltyCheckandSignalMatching/v2oVelocity_Plausibility/Plausibility_Test_SlipAngle ==
  Signal : Inport
  Signal_Sq : Inport  Port=2
  Bit Shift1 : hdlsllib/Logic and Bit Operations/Bit Shift  mode=Shift Left Logical  N=Sq_PosIsFrozen
      settings: SourceProductName=HDL Coder  SourceProductBaseCode=HD
  Bit Shift2 : hdlsllib/Logic and Bit Operations/Bit Shift  mode=Shift Left Logical  N=Sq_PosBadGradient
      settings: SourceProductName=HDL Coder  SourceProductBaseCode=HD
  Bit Shift3 : hdlsllib/Logic and Bit Operations/Bit Shift  mode=Shift Left Logical  N=Sq_PosOutOfBounds
      settings: SourceProductName=HDL Coder  SourceProductBaseCode=HD
  Bitwise Operator : simulink/Logic and Bit Operations/Bitwise Operator  logicop=OR  UseBitMask=off  NumInputPorts=4  BitMask=bin2dec('11011001')  BitMaskRealWorld=Stored Integer
  Constant : Constant  Value=checkGradient
  Constant1 : Constant  Value=useAlternativeValue
  Constant2 : Constant  Value=useManualAlternativeValue
  Constant3 : Constant  Value=manualAlternativeValue
  Data Type Conversion1 : DataTypeConversion  OutDataTypeStr=uint8
  Data Type Conversion2 : DataTypeConversion  OutDataTypeStr=uint8
  Data Type Conversion3 : DataTypeConversion  OutDataTypeStr=uint8
  If : If  IfExpression=u1 == 1  ShowElse=off
  If Action SignalQualifier_PlausibleGradient : Subsystem  TreatAsAtomicUnit=on
  Logical Operator : Logic  Operator=OR  Inputs=3  AllPortsSameDT=off  OutDataTypeStr=boolean
  Logical Operator1 : Logic  AllPortsSameDT=off  OutDataTypeStr=boolean
  Logical Operator2 : Logic  Operator=NOT  Inputs=1  AllPortsSameDT=off  OutDataTypeStr=boolean
  Rate Transition1 : RateTransition  OutPortSampleTime=0.004
  SignalQualifier_FrozenValue : Subsystem
  SignalQualifier_InBounds : Subsystem
  Switch : Switch  Criteria=u2 > Threshold
  Switch1 : Switch  Criteria=u2 > Threshold
  Switch2 : Switch  Criteria=u2 > Threshold
  Unit Delay : UnitDelay  SampleTime=-1
  lowpass : Subsystem
  Signal_out : Outport
  Signal_Sq_out : Outport  Port=2
  wires:
  Switch1/1 -> Switch2/3
  Logical Operator2/1 -> Switch2/2
  Logical Operator1/1 -> Logical Operator2/1
  Switch2/1 -> Signal_out/1
  Constant3/1 -> Switch1/1
  Constant2/1 -> Switch1/2
  Unit Delay/1 -> Switch/1, Switch1/3
  Switch/1 -> Unit Delay/1
  Constant1/1 -> Logical Operator1/1
  Logical Operator/1 -> Logical Operator1/2, Switch/2  "badSignal"
  Constant/1 -> If/1
  Data Type Conversion3/1 -> Bit Shift1/1
  Data Type Conversion2/1 -> Bit Shift3/1
  Data Type Conversion1/1 -> Bit Shift2/1
  Bit Shift2/1 -> Bitwise Operator/1
  Bitwise Operator/1 -> Signal_Sq_out/1
  If Action SignalQualifier_PlausibleGradient/1(BadGradient) -> Rate Transition1/1
  SignalQualifier_FrozenValue/1(IsFrozen) -> Data Type Conversion3/1, Logical Operator/3
  SignalQualifier_InBounds/1(IsOutOfBounds) -> Logical Operator/2, Data Type Conversion2/1
  Signal_Sq/1 -> Bitwise Operator/4
  Bit Shift3/1 -> Bitwise Operator/2
  Bit Shift1/1 -> Bitwise Operator/3
  lowpass/1(filtered signal) -> SignalQualifier_InBounds/1(FilteredSignal), If Action SignalQualifier_PlausibleGradient/2(filteredSignal), Switch/3
  Signal/1 -> lowpass/1(signal), If Action SignalQualifier_PlausibleGradient/1(Signal), Switch2/1, SignalQualifier_FrozenValue/1(signal)
  If/1 -> If Action SignalQualifier_PlausibleGradient/Action
  Rate Transition1/1 -> Logical Operator/1, Data Type Conversion1/1

== system vd_controller_E9/021_SignalProcessing/213_PlausibiltyCheckandSignalMatching/v2oVelocity_Plausibility/Plausibility_Test_SlipAngle/If Action SignalQualifier_PlausibleGradient ==
  Signal : Inport
  filteredSignal : Inport  Port=2
  Action Port : ActionPort  ActionType=then
  SignalQualifier_PlausibleGradient : Subsystem
  BadGradient : Outport
  wires:
  SignalQualifier_PlausibleGradient/1(BadGradient) -> BadGradient/1
  filteredSignal/1 -> SignalQualifier_PlausibleGradient/2(filteredSignal)
  Signal/1 -> SignalQualifier_PlausibleGradient/1(Signal)

== system vd_controller_E9/021_SignalProcessing/213_PlausibiltyCheckandSignalMatching/v2oVelocity_Plausibility/Plausibility_Test_SlipAngle/SignalQualifier_FrozenValue ==
  note: step delay:
      | how many steps must
      | the signal be within the
      | range, so that it is
      | detected as frozen
  note: bounds for signalchange
      | standard: 1e-6
  note: Counter which counts the steps, how long the signals are within the threshold
  note: Output
      | =1 if signal is frozen
      | =0 if signal is not frozen
  signal : Inport
  Abs1 : Abs
  Add1 : Sum  Inputs=+-
  Add3 : Sum
  Are the filtered signal and the normal signal near together? : simulink/Logic and Bit Operations/Compare To Constant  relop=<  const=signalBounds  OutDataTypeStr=boolean
  Compare To Constant1 : simulink/Logic and Bit Operations/Compare To Constant  relop=>  const=stepDelay  OutDataTypeStr=boolean
  Data Type Conversion1 : DataTypeConversion
  Data Type Conversion2 : DataTypeConversion
  Product1 : Product
  Unit Delay : UnitDelay  SampleTime=-1
  Unit Delay1 : UnitDelay  SampleTime=-1
  IsFrozen : Outport
  wires:
  signal/1 -> Add1/1, Unit Delay/1
  Product1/1 -> Data Type Conversion2/1, Compare To Constant1/1
  Unit Delay1/1 -> Add3/1
  Compare To Constant1/1 -> IsFrozen/1
  Abs1/1 -> Are the filtered signal and the normal signal near together?/1
  Add1/1 -> Abs1/1
  Unit Delay/1 -> Add1/2
  Are the filtered signal and the normal signal near together?/1 -> Data Type Conversion1/1
  Data Type Conversion1/1 -> Add3/2, Product1/2
  Data Type Conversion2/1 -> Unit Delay1/1
  Add3/1 -> Product1/1

== system vd_controller_E9/021_SignalProcessing/213_PlausibiltyCheckandSignalMatching/v2oVelocity_Plausibility/Plausibility_Test_SlipAngle/SignalQualifier_InBounds ==
  FilteredSignal : Inport
  Compare To Constant : simulink/Logic and Bit Operations/Compare To Constant  relop=>  const=upperBound  OutDataTypeStr=boolean
  Compare To Constant1 : simulink/Logic and Bit Operations/Compare To Constant  relop=<  const=lowerBound  OutDataTypeStr=boolean
  Logical Operator : Logic  Operator=OR  AllPortsSameDT=off  OutDataTypeStr=boolean
  IsOutOfBounds : Outport
  wires:
  FilteredSignal/1 -> Compare To Constant1/1, Compare To Constant/1
  Compare To Constant/1 -> Logical Operator/1
  Compare To Constant1/1 -> Logical Operator/2
  Logical Operator/1 -> IsOutOfBounds/1

== system vd_controller_E9/021_SignalProcessing/213_PlausibiltyCheckandSignalMatching/v2oVelocity_Plausibility/Plausibility_Test_SlipAngle/lowpass ==
  note: Lowpass_alpha is a parameter of the lowpass filter.
      | lowpass_alpha=1  --> no filtering (standard)
      | 0<lowpass_alpha<1   --> inertia of output signal
  signal : Inport
  Add1 : Sum  Inputs=-+
  Add2 : Sum
  Constant : Constant  Value=alpha
  Product : Product
  Unit Delay : UnitDelay  SampleTime=-1
  filtered signal : Outport
  wires:
  signal/1 -> Add1/2
  Add1/1 -> Product/1
  Add2/1 -> filtered signal/1, Unit Delay/1
  Unit Delay/1 -> Add1/1, Add2/1
  Constant/1 -> Product/2
  Product/1 -> Add2/2

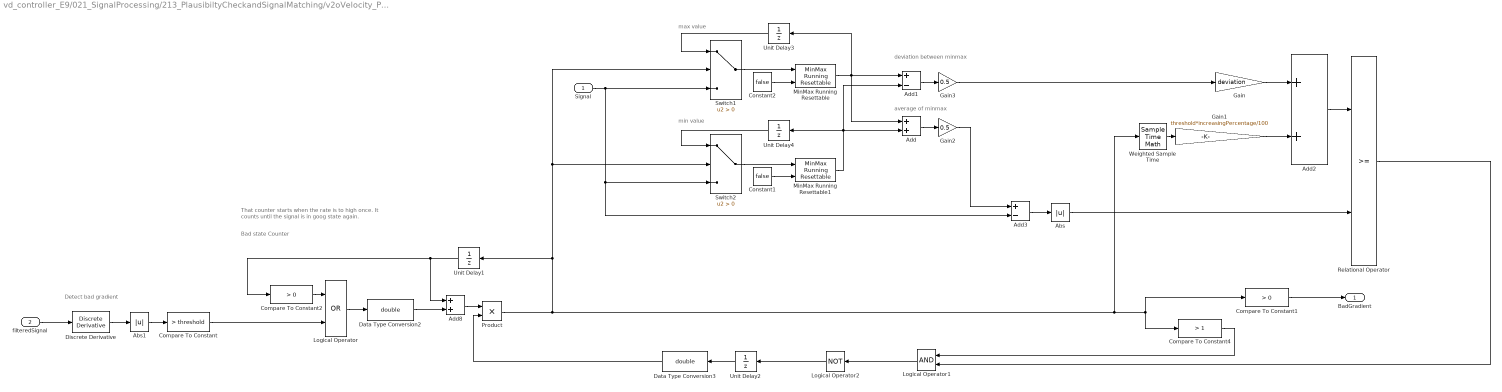
== system vd_controller_E9/021_SignalProcessing/213_PlausibiltyCheckandSignalMatching/v2oVelocity_Plausibility/Plausibility_Test_SlipAngle/If Action SignalQualifier_PlausibleGradient/SignalQualifier_PlausibleGradient ==
  note: Detect bad gradient
  note: That counter starts when the rate is to high once.
      | It counts until the signal is in goog state again.
  note: Bad state Counter
  note: max value
  note: min value
  note: average of minmax
  note: deviation between minmax
  Signal : Inport
  filteredSignal : Inport  Port=2
  Abs : Abs
  Abs1 : Abs
  Add : Sum
  Add1 : Sum  Inputs=+-
  Add2 : Sum
  Add3 : Sum  Inputs=+-
  Add8 : Sum  AccumDataTypeStr=double  OutDataTypeStr=double
  Compare To Constant : simulink/Logic and Bit Operations/Compare To Constant  relop=>  const=threshold  OutDataTypeStr=boolean
  Compare To Constant1 : simulink/Logic and Bit Operations/Compare To Constant  relop=>  const=0  OutDataTypeStr=boolean
  Compare To Constant2 : simulink/Logic and Bit Operations/Compare To Constant  relop=>  const=0  OutDataTypeStr=boolean
  Compare To Constant4 : simulink/Logic and Bit Operations/Compare To Constant  relop=>  const=1  OutDataTypeStr=boolean
  Constant1 : Constant  Value=false
  Constant2 : Constant  Value=false
  Data Type Conversion2 : DataTypeConversion  OutDataTypeStr=double
  Data Type Conversion3 : DataTypeConversion  OutDataTypeStr=double
  Discrete Derivative : simulink/Discrete/Discrete Derivative  gainval=1.0  ICPrevScaledInput=0.0  OutMin=[]  OutMax=[]  OutDataType=fixdt(1, 16)  OutScaling=2^-10  DoSatur=off
  Gain : Gain  Gain=deviation
  Gain1 : Gain  Gain=threshold*increasingPercentage/100
  Gain2 : Gain  Gain=0.5
  Gain3 : Gain  Gain=0.5
  Logical Operator : Logic  Operator=OR  AllPortsSameDT=off  OutDataTypeStr=boolean
  Logical Operator1 : Logic  AllPortsSameDT=off  OutDataTypeStr=boolean
  Logical Operator2 : Logic  Operator=NOT  AllPortsSameDT=off  OutDataTypeStr=boolean
  MinMax Running Resettable : simulink/Math Operations/MinMax Running Resettable  Function=max  vinit=0.0
  MinMax Running Resettable1 : simulink/Math Operations/MinMax Running Resettable  Function=min  vinit=0.0
  Product : Product  OutDataTypeStr=double
  Relational Operator : RelationalOperator  OutDataTypeStr=boolean  RndMeth=Simplest
  Switch1 : Switch  Criteria=u2 > Threshold
  Switch2 : Switch  Criteria=u2 > Threshold
  Unit Delay{1..4} (4 alike) : UnitDelay  SampleTime=-1
  Weighted Sample Time : SampleTimeMath  TsampMathOp=*
  BadGradient : Outport
  wires:
  Unit Delay4/1 -> Switch2/1
  Unit Delay3/1 -> Switch1/1
  Abs/1 -> Relational Operator/2
  Add3/1 -> Abs/1
  Gain2/1 -> Add3/1
  Gain3/1 -> Gain/1
  Add1/1 -> Gain3/1
  Add/1 -> Gain2/1
  MinMax Running Resettable1/1 -> Add/2, Unit Delay4/1, Add1/2
  Switch2/1 -> MinMax Running Resettable1/1
  Constant1/1 -> MinMax Running Resettable1/2
  Constant2/1 -> MinMax Running Resettable/2
  MinMax Running Resettable/1 -> Unit Delay3/1, Add1/1, Add/1
  Switch1/1 -> MinMax Running Resettable/1
  Discrete Derivative/1 -> Abs1/1
  filteredSignal/1 -> Discrete Derivative/1
  Abs1/1 -> Compare To Constant/1
  Compare To Constant/1 -> Logical Operator/2
  Product/1 -> Compare To Constant1/1, Compare To Constant4/1, Weighted Sample Time/1, Unit Delay1/1, Switch2/2, Switch1/2
  Compare To Constant1/1 -> BadGradient/1
  Logical Operator/1 -> Data Type Conversion2/1
  Compare To Constant2/1 -> Logical Operator/1
  Gain/1 -> Add2/1
  Gain1/1 -> Add2/2
  Add2/1 -> Relational Operator/1
  Relational Operator/1 -> Logical Operator1/2
  Logical Operator1/1 -> Logical Operator2/1
  Add8/1 -> Product/1
  Data Type Conversion2/1 -> Add8/2
  Data Type Conversion3/1 -> Product/2
  Signal/1 -> Switch1/3, Add3/2, Switch2/3
  Logical Operator2/1 -> Unit Delay2/1
  Unit Delay1/1 -> Compare To Constant2/1, Add8/1
  Unit Delay2/1 -> Data Type Conversion3/1
  Compare To Constant4/1 -> Logical Operator1/1
  Weighted Sample Time/1 -> Gain1/1

== matlab function vd_controller_E9/024a_TractionControlForMinimal/LyapControl1/LyapControl ==
  data: v input; kappav_diff output; dotv input; omega input; Fz input; kappa_soll input; T output; Lyap_p parameter; velLimitInput input; tire_r_dyn parameter; WheelInertia parameter; Fz0 parameter; p_Dx1 parameter; p_Dx2 parameter; kappa output; Lyap_kp input; lambda_mux input
function [kappav_diff, T, kappa] = TC(v, dotv, omega, Fz, kappa_soll, Lyap_p,velLimitInput, tire_r_dyn, WheelInertia, Fz0, p_Dx1, p_Dx2, Lyap_kp, lambda_mux)
%#codegen

velLimit= velLimitInput;

% Schlupfgeschwindigkeitsberechnung
kappav_soll = kappa_soll.*v;
for i = 1:4
    if v(i)<velLimit
    kappav_soll(i) = kappa_soll(i)*velLimit;
    end
end
kappav = omega*tire_r_dyn - v;
kappa = kappav./v;
kappav_diff = kappav_soll - kappav; % = Regelgröße

% Pacejka
dfz = (Fz-Fz0)/Fz0;
mu_x = (p_Dx1 + p_Dx2*dfz)*lambda_mux;
D_x = mu_x.*Fz;
 
% Reglergesetz
T = WheelInertia/tire_r_dyn*((1+kappa_soll).*dotv+tire_r_dyn^2/WheelInertia*abs(D_x).*sign(kappav_soll)+Lyap_kp*kappav_diff.^Lyap_p);

%Filterwerte davor 0.02 -0,98
%Sinnvolle Werte für -0.95 bis 0.9 wird glatter / träger

== matlab function vd_controller_E9/024a_TractionControlForMinimal/LyapControl1/MATLAB Function ==
  data: num output; den output; LyapDiscFilter input
function [num,den] = filterCoeffs(LyapDiscFilter)

num = 1 + LyapDiscFilter;
den = [1 LyapDiscFilter];
